simulink model "Five_level_MCI_PMSM_Control_1_fault_tolerant"  (R2025a)
settings: Solver=VariableStepAuto  StartTime=0.0  StopTime=13  RelTol=1e-3
undefined symbols (not defined in the file or in its folder): Ion, Lithium
libraries: spsIGBTDiodeLib x24, spsCurrentMeasurementLib x12, spsVoltageMeasurementLib x6, spsBatteryLib x6, spsRMSLib x6, spsBreakerLib x4, slpidlib x1, spsGroundLib x1, spsPermanentMagnetSynchronousMachineLib x1, simulink x1, spsThreePhaseVIMeasurementLib x1, sps_lib x1
settings Model: Creator=mugun  LastModifiedBy=mugun

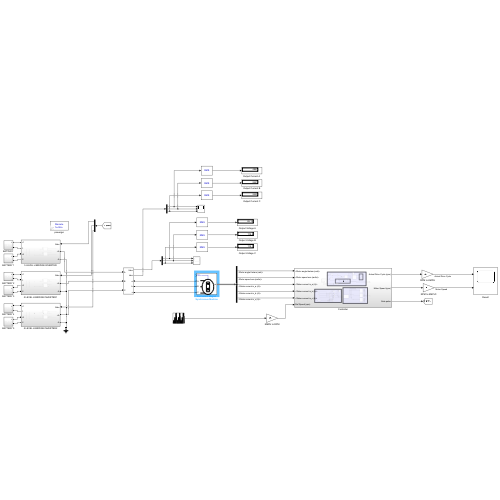
[thumbnail: Simulink's stored preview of the top-level diagram]
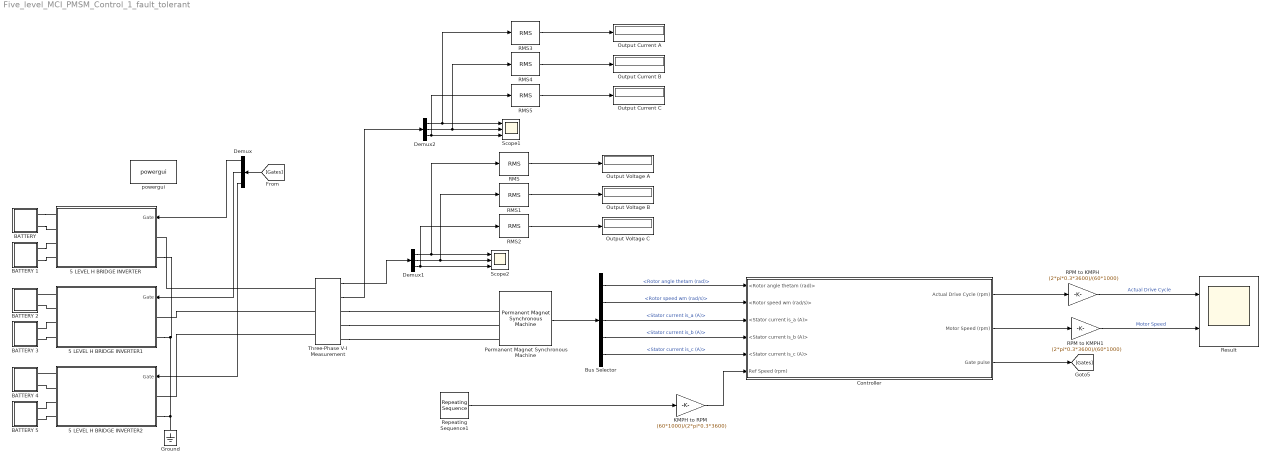
== system Five_level_MCI_PMSM_Control_1_fault_tolerant ==
  5 LEVEL H BRIDGE INVERTER : Subsystem
      settings: PortSchema="{\"entries\":[{\"content\":{\"sides\":[{\"content\":{\"connectorIds\":[\"LConn1\",\"LConn2\",\"LConn3\",\"LConn4\"]},\"type\":\"ConnectorPlacement.EquallySpacedRectSide\",\"uuid\":\"a99ba5a4-868b-4ca9-ae89-158e30df76de\"},{\"content\":{\"connectorIds\":[\"In1\",\"RConn1\",\"RConn2\"],\"side\":\"RIGHT\"},\"type\":\"ConnectorPlacement.EquallySpacedRectSide\",\"uuid\":\"907b6b32-6b28-4f9b-aa63-058c17a50e82\"},{\"content\":{\"side\":\"TOP\"},\"type\":\"ConnectorPlacement.EquallySpacedRectSide\",\"uuid\":\"64bd340d-5502-4b77-92cb-0ed146f38aa8\"}]},\"type\":\"ConnectorPlacement.EquallySpacedConnector\",\"uuid\":\"1fa2cca1-805b-4996-9e9c-123ddddb2b33\"}],\"packageUris\":[\"http://schema.mathworks.com/mf0/Connector/R2020b\"],\"version\":\"1.0\"}"
  5 LEVEL H BRIDGE INVERTER1 : Subsystem
      settings: PortSchema="{\"entries\":[{\"content\":{\"sides\":[{\"content\":{\"connectorIds\":[\"LConn1\",\"LConn2\",\"LConn3\",\"LConn4\"]},\"type\":\"ConnectorPlacement.EquallySpacedRectSide\",\"uuid\":\"a99ba5a4-868b-4ca9-ae89-158e30df76de\"},{\"content\":{\"connectorIds\":[\"In1\",\"RConn1\",\"RConn2\"],\"side\":\"RIGHT\"},\"type\":\"ConnectorPlacement.EquallySpacedRectSide\",\"uuid\":\"907b6b32-6b28-4f9b-aa63-058c17a50e82\"},{\"content\":{\"side\":\"TOP\"},\"type\":\"ConnectorPlacement.EquallySpacedRectSide\",\"uuid\":\"64bd340d-5502-4b77-92cb-0ed146f38aa8\"}]},\"type\":\"ConnectorPlacement.EquallySpacedConnector\",\"uuid\":\"1fa2cca1-805b-4996-9e9c-123ddddb2b33\"}],\"packageUris\":[\"http://schema.mathworks.com/mf0/Connector/R2020b\"],\"version\":\"1.0\"}"
  5 LEVEL H BRIDGE INVERTER2 : Subsystem
      settings: PortSchema="{\"entries\":[{\"content\":{\"sides\":[{\"content\":{\"connectorIds\":[\"LConn1\",\"LConn2\",\"LConn3\",\"LConn4\"]},\"type\":\"ConnectorPlacement.EquallySpacedRectSide\",\"uuid\":\"a99ba5a4-868b-4ca9-ae89-158e30df76de\"},{\"content\":{\"connectorIds\":[\"In1\",\"RConn1\",\"RConn2\"],\"side\":\"RIGHT\"},\"type\":\"ConnectorPlacement.EquallySpacedRectSide\",\"uuid\":\"907b6b32-6b28-4f9b-aa63-058c17a50e82\"},{\"content\":{\"side\":\"TOP\"},\"type\":\"ConnectorPlacement.EquallySpacedRectSide\",\"uuid\":\"64bd340d-5502-4b77-92cb-0ed146f38aa8\"}]},\"type\":\"ConnectorPlacement.EquallySpacedConnector\",\"uuid\":\"1fa2cca1-805b-4996-9e9c-123ddddb2b33\"}],\"packageUris\":[\"http://schema.mathworks.com/mf0/Connector/R2020b\"],\"version\":\"1.0\"}"
  "BATTERY " : Subsystem
  BATTERY 1 : Subsystem
  BATTERY 2 : Subsystem
  BATTERY 3 : Subsystem
  BATTERY 4 : Subsystem
  BATTERY 5 : Subsystem
  Bus Selector : BusSelector  OutputSignals=Rotor angle thetam (rad),Rotor speed wm (rad/s),Stator current is_a (A),Stator current is_b (A),Stator current is_c (A)
  Controller : Subsystem
  Demux : Demux  Outputs=3
  Demux1 : Demux  Outputs=3
  Demux2 : Demux  Outputs=3
  Ground : spsGroundLib/Ground  LConnTagsString=a
  KMPH to RPM : Gain  Gain=(60*1000)/(2*pi*0.3*3600)
  "Output Current A " : Display
  Output Current B : Display
  Output Current C : Display
  Output Voltage A : Display
  Output Voltage B : Display
  Output Voltage C : Display
  Permanent Magnet Synchronous Machine : spsPermanentMagnetSynchronousMachineLib/Permanent Magnet Synchronous Machine  NbPhases=3  FluxDistribution=Sinusoidal  RotorType=Round  MechanicalLoad=Torque Tm  PresetModel=No  ShowDetailedParameters=on  MeasurementBus=off  Resistance=0.02  Inductance=8.5e-3  dqInductances=[8.5e-3,8.5e-3]  La=0.00025  MachineConstant=Flux linkage established by magnets (V.s)  Flux=0.133833  VoltageCst=97.0985  TorqueCst=0.803  Flat=120  Mechanical=[0.008 0.003 4]  PolePairs=4  InitialConditions=[0,0, 0,0]  InitialConditions5ph=[0 0 0 0 0 0]  RefAngle=90 degrees behind phase A axis (modified Park)  IterativeDiscreteModel=Trapezoidal non iterative  TsBlock=-1  TsPowergui=0
  RMS{,1..5} (6 alike) : spsRMSLib/RMS  TrueRMS=on  Freq=60  RMSInit=120  Ts=0
  RPM to KMPH : Gain  Gain=(2*pi*0.3*3600)/(60*1000)
  RPM to KMPH1 : Gain  Gain=(2*pi*0.3*3600)/(60*1000)
  Repeating Sequence1 : simulink/Sources/Repeating Sequence  rep_seq_t=[0 1 2 3 4 5 6 7 8 9 10 11 11.0001 12 13]  rep_seq_y=[0 0 10 10 0 0 20 20 0 0 35 35 25 25 0]
  Result : Scope  NumInputPorts=2
      settings: ActiveDisplayYMinimum=-1  ActiveDisplayYMaximum=1  DataLoggingVariableName=ScopeData8
  Scope1 : Scope  NumInputPorts=3
      settings: ActiveDisplayYMinimum=-1.0013001136517929  ActiveDisplayYMaximum=1.1229859234420478
  Scope2 : Scope  NumInputPorts=3
      settings: ActiveDisplayYMinimum=-132.61800974908385  ActiveDisplayYMaximum=132.61868398150364  DataLoggingVariableName=ScopeData9
  Three-Phase V-I Measurement : spsThreePhaseVIMeasurementLib/Three-Phase V-I Measurement  VoltageMeasurement=phase-to-ground  SetLabelV=off  LabelV=Vabc  Vpu=off  VpuLL=off  CurrentMeasurement=yes  SetLabelI=off  LabelI=Iabc  Ipu=off  Pbase=100e6  Vbase=500e3  OutputType=Complex  PhasorSimulation=off  PSBequivalent=0
  powergui : sps_lib/powergui  Priority=1  SimulationMode=Discrete  SampleTime=1e-6  frequency=60  Iterations=50  frequencyindice=0  Pbase=100e6  ErrMax=1e-4  UnitsV=kV  UnitsW=MW  buscounter=0  FunctionMessages=off  echomessages=off  EnableUseOfTLC=off  CurrentSourceSwitches=off  DisableSnubberDevices=off  DisableRonSwitches=off  DisableVfSwitches=off  DisplayEquations=off  AutomaticDiscreteSolvers=off  SolverType=Tustin/Backward Euler (TBE)  Interpol=off  ExternalGateDelay=off  methode=off  Ts=100  x0status=blocks  SPID=on  SwTol=0  HookPort=off  NonlinearTolerance=1e-4  nMaxIteration=100  ContinueOnMaxIteration=off  RestoreLinks=warning  ResistiveCurrentMeasurement=off  Frange=[0:2:500]  Ylog=off  Xlog=on  ShowGrid=off  save=off  variable=ZData  structure=0  ZoomFFT=off  StartTime=0.0  cycles=1  DisplayStyle=1  fundamental=60  FreqAxis=off  MaxFrequency=1000  frequencyindicesteady=1  RmsSteady=1  display=off
  wires:
  RMS2/1 -> Output Voltage C/1
  KMPH to RPM/1 -> Controller/6(Ref Speed (rpm))
  Bus Selector/3 -> Controller/3(<Stator current is_a (A)>)  "<Stator current is_a (A)>"
  Demux1/1 -> RMS/1, Scope2/1
  Three-Phase V-I Measurement/1 -> Demux1/1
  Demux1/2 -> RMS1/1, Scope2/2
  Demux1/3 -> RMS2/1, Scope2/3
  RMS/1 -> Output Voltage A/1
  Permanent Magnet Synchronous Machine/1 -> Bus Selector/1
  Bus Selector/2 -> Controller/2(<Rotor speed wm (rad/s)>)  "<Rotor speed wm (rad/s)>"
  Bus Selector/4 -> Controller/4(<Stator current is_b (A)>)  "<Stator current is_b (A)>"
  RMS1/1 -> Output Voltage B/1
  Controller/3(Gate pulse) -> [Gates]
  Controller/2(Motor Speed (rpm)) -> RPM to KMPH1/1
  Controller/1(Actual Drive Cycle (rpm)) -> RPM to KMPH/1
  Bus Selector/1 -> Controller/1(<Rotor angle thetam (rad)>)  "<Rotor angle thetam (rad)>"
  Bus Selector/5 -> Controller/5(<Stator current is_c (A)>)  "<Stator current is_c (A)>"
  Demux/1 -> 5 LEVEL H BRIDGE INVERTER/1(Gate)
  Demux/2 -> 5 LEVEL H BRIDGE INVERTER1/1(Gate)
  Demux/3 -> 5 LEVEL H BRIDGE INVERTER2/1(Gate)
  [Gates] -> Demux/1
  RPM to KMPH/1 -> Result/1  "Actual Drive Cycle"
  RPM to KMPH1/1 -> Result/2  "Motor Speed"
  Repeating Sequence1/1 -> KMPH to RPM/1
  RMS3/1 -> "Output Current A "/1
  RMS4/1 -> Output Current B/1
  Demux2/2 -> RMS4/1, Scope1/2
  Demux2/1 -> RMS3/1, Scope1/1
  Demux2/3 -> RMS5/1, Scope1/3
  Three-Phase V-I Measurement/2 -> Demux2/1
  RMS5/1 -> Output Current C/1
  connections:
  Three-Phase V-I Measurement/RConn2 -- Permanent Magnet Synchronous Machine/LConn2
  Three-Phase V-I Measurement/RConn1 -- Permanent Magnet Synchronous Machine/LConn1
  Three-Phase V-I Measurement/RConn3 -- Permanent Magnet Synchronous Machine/LConn3
  Ground/LConn1 -- 5 LEVEL H BRIDGE INVERTER/RConn2 -- 5 LEVEL H BRIDGE INVERTER1/RConn2 -- 5 LEVEL H BRIDGE INVERTER2/RConn2
  5 LEVEL H BRIDGE INVERTER2/LConn4 -- BATTERY 5/LConn2
  5 LEVEL H BRIDGE INVERTER1/LConn1 -- BATTERY 2/LConn1
  5 LEVEL H BRIDGE INVERTER2/LConn1 -- BATTERY 4/LConn1
  BATTERY 1/LConn2 -- 5 LEVEL H BRIDGE INVERTER/LConn4
  5 LEVEL H BRIDGE INVERTER2/LConn3 -- BATTERY 5/LConn1
  5 LEVEL H BRIDGE INVERTER1/LConn3 -- BATTERY 3/LConn1
  5 LEVEL H BRIDGE INVERTER2/LConn2 -- BATTERY 4/LConn2
  Three-Phase V-I Measurement/LConn2 -- 5 LEVEL H BRIDGE INVERTER1/RConn1
  Three-Phase V-I Measurement/LConn3 -- 5 LEVEL H BRIDGE INVERTER2/RConn1
  5 LEVEL H BRIDGE INVERTER1/LConn4 -- BATTERY 3/LConn2
  Three-Phase V-I Measurement/LConn1 -- 5 LEVEL H BRIDGE INVERTER/RConn1
  "BATTERY "/LConn1 -- 5 LEVEL H BRIDGE INVERTER/LConn1
  5 LEVEL H BRIDGE INVERTER1/LConn2 -- BATTERY 2/LConn2
  BATTERY 1/LConn1 -- 5 LEVEL H BRIDGE INVERTER/LConn3
  "BATTERY "/LConn2 -- 5 LEVEL H BRIDGE INVERTER/LConn2

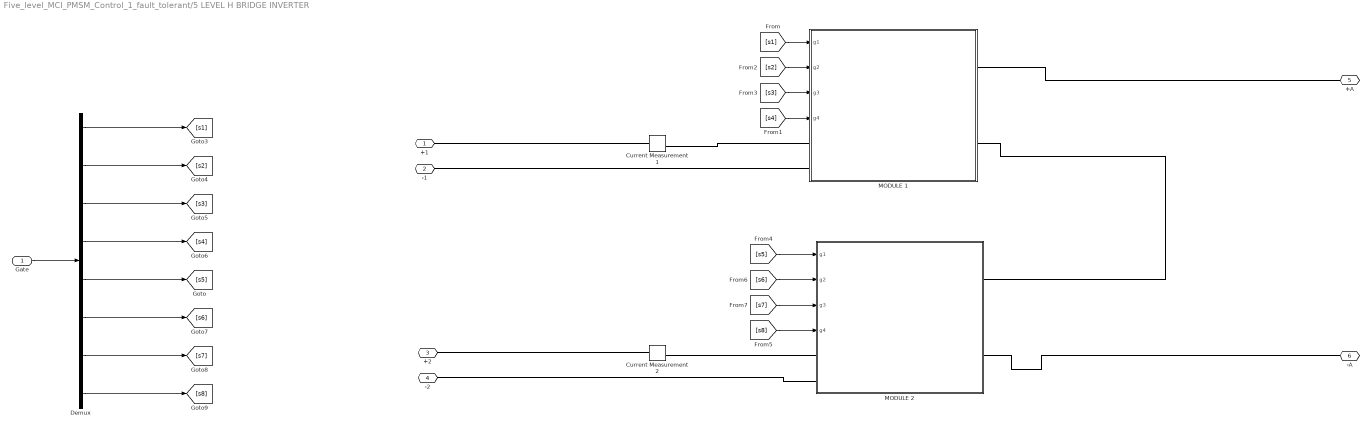
== system Five_level_MCI_PMSM_Control_1_fault_tolerant/5 LEVEL H BRIDGE INVERTER ==
  Gate : Inport
  Current Measurement1 : spsCurrentMeasurementLib/Current Measurement  PhasorSimulation=off  OutputType=Complex  PSBequivalent=0
  Current Measurement2 : spsCurrentMeasurementLib/Current Measurement  PhasorSimulation=off  OutputType=Complex  PSBequivalent=0
  Demux : Demux  Outputs=8
  MODULE 1 : Subsystem
  MODULE 2 : Subsystem
  +1 : PMIOPort  Side=Left
  -1 : PMIOPort  Port=2  Side=Left
  +2 : PMIOPort  Port=3  Side=Left
  -2 : PMIOPort  Port=4  Side=Left
  +A : PMIOPort  Port=5  Side=Right
  -A : PMIOPort  Port=6  Side=Right
  wires:
  Demux/1 -> [s1]
  Demux/2 -> [s2]
  Demux/3 -> [s3]
  Demux/4 -> [s4]
  Demux/5 -> [s5]
  Demux/6 -> [s6]
  Demux/7 -> [s7]
  Demux/8 -> [s8]
  Gate/1 -> Demux/1
  [s3] -> MODULE 1/3(g3)
  [s1] -> MODULE 1/1(g1)
  [s4] -> MODULE 1/4(g4)
  [s2] -> MODULE 1/2(g2)
  [s6] -> MODULE 2/2(g2)
  [s8] -> MODULE 2/4(g4)
  [s5] -> MODULE 2/1(g1)
  [s7] -> MODULE 2/3(g3)
  connections:
  +1/RConn1 -- Current Measurement1/LConn1
  Current Measurement1/RConn1 -- MODULE 1/LConn1
  -1/RConn1 -- MODULE 1/LConn2
  Current Measurement2/RConn1 -- MODULE 2/LConn1
  -2/RConn1 -- MODULE 2/LConn2
  +2/RConn1 -- Current Measurement2/LConn1
  MODULE 1/RConn1 -- +A/RConn1
  MODULE 1/RConn2 -- MODULE 2/RConn1
  MODULE 2/RConn2 -- -A/RConn1

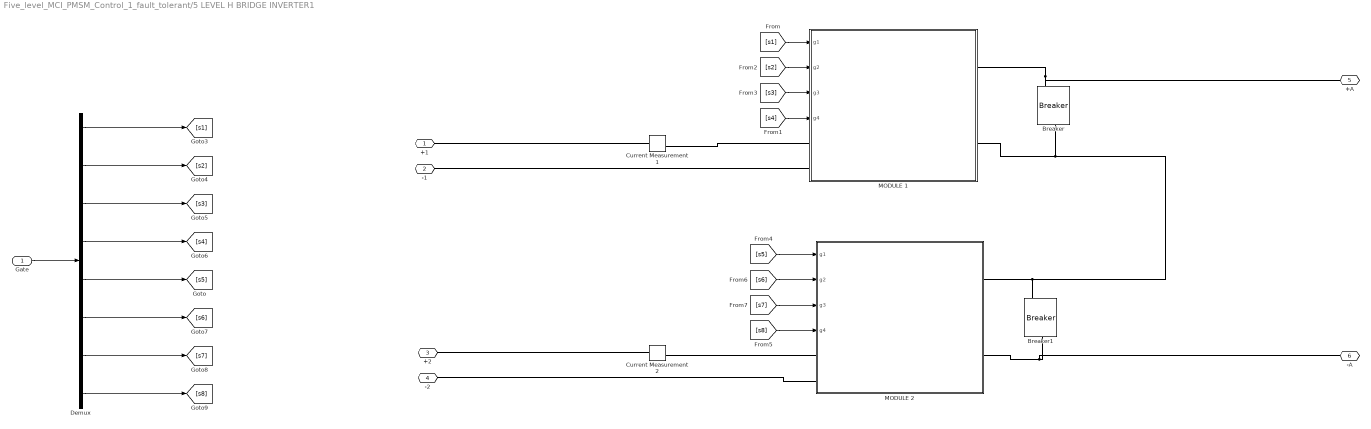
== system Five_level_MCI_PMSM_Control_1_fault_tolerant/5 LEVEL H BRIDGE INVERTER1 ==
  Gate : Inport
  Breaker : spsBreakerLib/Breaker  InitialState=0  SwitchingTimes="[1/60  5/60]"  External=on  BreakerResistance=0.01  SnubberResistance=1e10  SnubberCapacitance=inf  Measurements=None  MoreParameters=on  NoBreakLoop=off
  Breaker1 : spsBreakerLib/Breaker  InitialState=0  SwitchingTimes="[1/60  5/60]"  External=on  BreakerResistance=0.01  SnubberResistance=1e10  SnubberCapacitance=inf  Measurements=None  MoreParameters=on  NoBreakLoop=off
  Current Measurement1 : spsCurrentMeasurementLib/Current Measurement  PhasorSimulation=off  OutputType=Complex  PSBequivalent=0
  Current Measurement2 : spsCurrentMeasurementLib/Current Measurement  PhasorSimulation=off  OutputType=Complex  PSBequivalent=0
  Demux : Demux  Outputs=8
  MODULE 1 : Subsystem
  MODULE 2 : Subsystem
  +1 : PMIOPort  Side=Left
  -1 : PMIOPort  Port=2  Side=Left
  +2 : PMIOPort  Port=3  Side=Left
  -2 : PMIOPort  Port=4  Side=Left
  +A : PMIOPort  Port=5  Side=Right
  -A : PMIOPort  Port=6  Side=Right
  wires:
  Demux/1 -> [s1]
  Demux/2 -> [s2]
  Demux/3 -> [s3]
  Demux/4 -> [s4]
  Demux/5 -> [s5]
  Demux/6 -> [s6]
  Demux/7 -> [s7]
  Demux/8 -> [s8]
  Gate/1 -> Demux/1
  [s3] -> MODULE 1/3(g3)
  [s1] -> MODULE 1/1(g1)
  [s4] -> MODULE 1/4(g4)
  [s2] -> MODULE 1/2(g2)
  [s6] -> MODULE 2/2(g2)
  [s8] -> MODULE 2/4(g4)
  [s5] -> MODULE 2/1(g1)
  [s7] -> MODULE 2/3(g3)
  connections:
  +1/RConn1 -- Current Measurement1/LConn1
  Current Measurement1/RConn1 -- MODULE 1/LConn1
  -1/RConn1 -- MODULE 1/LConn2
  Current Measurement2/RConn1 -- MODULE 2/LConn1
  -2/RConn1 -- MODULE 2/LConn2
  +2/RConn1 -- Current Measurement2/LConn1
  Breaker/RConn1 -- MODULE 1/RConn2 -- MODULE 2/RConn1 -- Breaker1/LConn1
  Breaker1/RConn1 -- -A/RConn1 -- MODULE 2/RConn2
  MODULE 1/RConn1 -- Breaker/LConn1 -- +A/RConn1

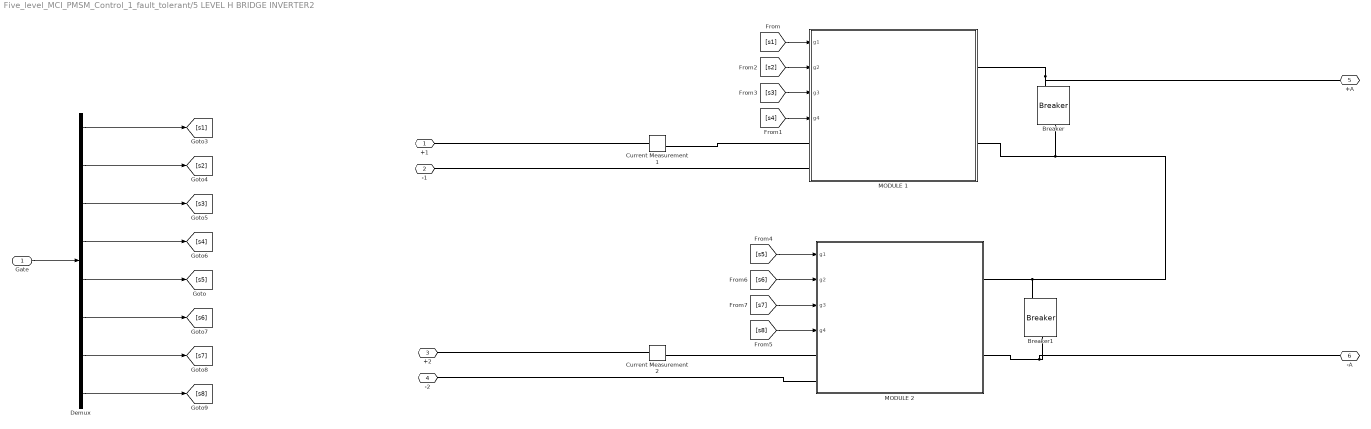
== system Five_level_MCI_PMSM_Control_1_fault_tolerant/5 LEVEL H BRIDGE INVERTER2 ==
  Gate : Inport
  Breaker : spsBreakerLib/Breaker  InitialState=0  SwitchingTimes="[1/60  5/60]"  External=on  BreakerResistance=0.01  SnubberResistance=1e10  SnubberCapacitance=inf  Measurements=None  MoreParameters=on  NoBreakLoop=off
  Breaker1 : spsBreakerLib/Breaker  InitialState=0  SwitchingTimes="[1/60  5/60]"  External=on  BreakerResistance=0.01  SnubberResistance=1e10  SnubberCapacitance=inf  Measurements=None  MoreParameters=on  NoBreakLoop=off
  Current Measurement1 : spsCurrentMeasurementLib/Current Measurement  PhasorSimulation=off  OutputType=Complex  PSBequivalent=0
  Current Measurement2 : spsCurrentMeasurementLib/Current Measurement  PhasorSimulation=off  OutputType=Complex  PSBequivalent=0
  Demux : Demux  Outputs=8
  MODULE 1 : Subsystem
  MODULE 2 : Subsystem
  +1 : PMIOPort  Side=Left
  -1 : PMIOPort  Port=2  Side=Left
  +2 : PMIOPort  Port=3  Side=Left
  -2 : PMIOPort  Port=4  Side=Left
  +A : PMIOPort  Port=5  Side=Right
  -A : PMIOPort  Port=6  Side=Right
  wires:
  Demux/1 -> [s1]
  Demux/2 -> [s2]
  Demux/3 -> [s3]
  Demux/4 -> [s4]
  Demux/5 -> [s5]
  Demux/6 -> [s6]
  Demux/7 -> [s7]
  Demux/8 -> [s8]
  Gate/1 -> Demux/1
  [s3] -> MODULE 1/3(g3)
  [s1] -> MODULE 1/1(g1)
  [s4] -> MODULE 1/4(g4)
  [s2] -> MODULE 1/2(g2)
  [s6] -> MODULE 2/2(g2)
  [s8] -> MODULE 2/4(g4)
  [s5] -> MODULE 2/1(g1)
  [s7] -> MODULE 2/3(g3)
  connections:
  +1/RConn1 -- Current Measurement1/LConn1
  Current Measurement1/RConn1 -- MODULE 1/LConn1
  -1/RConn1 -- MODULE 1/LConn2
  Current Measurement2/RConn1 -- MODULE 2/LConn1
  -2/RConn1 -- MODULE 2/LConn2
  +2/RConn1 -- Current Measurement2/LConn1
  Breaker/RConn1 -- MODULE 1/RConn2 -- MODULE 2/RConn1 -- Breaker1/LConn1
  Breaker1/RConn1 -- -A/RConn1 -- MODULE 2/RConn2
  MODULE 1/RConn1 -- Breaker/LConn1 -- +A/RConn1

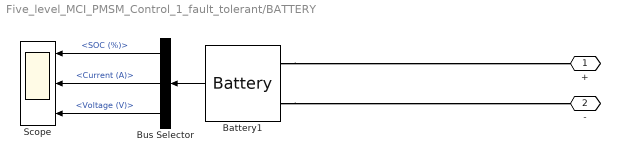
== system Five_level_MCI_PMSM_Control_1_fault_tolerant/BATTERY  ==
  Battery1 : spsBatteryLib/Battery  BatType=Lithium-Ion  NomV=98  NomQ=110  SOC=80  Batt_Tr=0.1  PresetModel=on  MaxQ=110  MinV=73.5  FullV=114.0707  Dis_rate=47.8261  R=0.0089091  Normal_OP=99.4783  expZone="[105.8778      5.404348]"
  Bus Selector : BusSelector  OutputSignals=SOC (%),Current (A),Voltage (V)
  Scope : Scope  NumInputPorts=3
      settings: ActiveDisplayYMinimum=80.6576402320921  ActiveDisplayYMaximum=80.657640232110069
  + : PMIOPort  Side=Left
  - : PMIOPort  Port=2  Side=Left
  wires:
  Bus Selector/3 -> Scope/3  "<Voltage (V)>"
  Battery1/1 -> Bus Selector/1
  Bus Selector/2 -> Scope/2  "<Current (A)>"
  Bus Selector/1 -> Scope/1  "<SOC (%)>"
  connections:
  Battery1/LConn2 -- -/RConn1
  Battery1/LConn1 -- +/RConn1

== system Five_level_MCI_PMSM_Control_1_fault_tolerant/BATTERY 1 ==
  Battery1 : spsBatteryLib/Battery  BatType=Lithium-Ion  NomV=98  NomQ=110  SOC=80  Batt_Tr=0.1  PresetModel=on  MaxQ=110  MinV=73.5  FullV=114.0707  Dis_rate=47.8261  R=0.0089091  Normal_OP=99.4783  expZone="[105.8778      5.404348]"
  Bus Selector : BusSelector  OutputSignals=SOC (%),Current (A),Voltage (V)
  Scope : Scope  NumInputPorts=3
      settings: ActiveDisplayYMinimum=80.6576402320921  ActiveDisplayYMaximum=80.657640232110069
  + : PMIOPort  Side=Left
  - : PMIOPort  Port=2  Side=Left
  wires:
  Bus Selector/3 -> Scope/3  "<Voltage (V)>"
  Battery1/1 -> Bus Selector/1
  Bus Selector/2 -> Scope/2  "<Current (A)>"
  Bus Selector/1 -> Scope/1  "<SOC (%)>"
  connections:
  Battery1/LConn2 -- -/RConn1
  Battery1/LConn1 -- +/RConn1

== system Five_level_MCI_PMSM_Control_1_fault_tolerant/BATTERY 2 ==
  Battery1 : spsBatteryLib/Battery  BatType=Lithium-Ion  NomV=98  NomQ=110  SOC=80  Batt_Tr=0.1  PresetModel=on  MaxQ=110  MinV=73.5  FullV=114.0707  Dis_rate=47.8261  R=0.0089091  Normal_OP=99.4783  expZone="[105.8778      5.404348]"
  Bus Selector : BusSelector  OutputSignals=SOC (%),Current (A),Voltage (V)
  Scope : Scope  NumInputPorts=3
      settings: ActiveDisplayYMinimum=80.6576402320921  ActiveDisplayYMaximum=80.657640232110069
  + : PMIOPort  Side=Left
  - : PMIOPort  Port=2  Side=Left
  wires:
  Bus Selector/3 -> Scope/3  "<Voltage (V)>"
  Battery1/1 -> Bus Selector/1
  Bus Selector/2 -> Scope/2  "<Current (A)>"
  Bus Selector/1 -> Scope/1  "<SOC (%)>"
  connections:
  Battery1/LConn2 -- -/RConn1
  Battery1/LConn1 -- +/RConn1

== system Five_level_MCI_PMSM_Control_1_fault_tolerant/BATTERY 3 ==
  Battery1 : spsBatteryLib/Battery  BatType=Lithium-Ion  NomV=98  NomQ=110  SOC=80  Batt_Tr=0.1  PresetModel=on  MaxQ=110  MinV=73.5  FullV=114.0707  Dis_rate=47.8261  R=0.0089091  Normal_OP=99.4783  expZone="[105.8778      5.404348]"
  Bus Selector : BusSelector  OutputSignals=SOC (%),Current (A),Voltage (V)
  Scope : Scope  NumInputPorts=3
      settings: ActiveDisplayYMinimum=80.6576402320921  ActiveDisplayYMaximum=80.657640232110069
  + : PMIOPort  Side=Left
  - : PMIOPort  Port=2  Side=Left
  wires:
  Bus Selector/3 -> Scope/3  "<Voltage (V)>"
  Battery1/1 -> Bus Selector/1
  Bus Selector/2 -> Scope/2  "<Current (A)>"
  Bus Selector/1 -> Scope/1  "<SOC (%)>"
  connections:
  Battery1/LConn2 -- -/RConn1
  Battery1/LConn1 -- +/RConn1

== system Five_level_MCI_PMSM_Control_1_fault_tolerant/BATTERY 4 ==
  Battery1 : spsBatteryLib/Battery  BatType=Lithium-Ion  NomV=98  NomQ=110  SOC=80  Batt_Tr=0.1  PresetModel=on  MaxQ=110  MinV=73.5  FullV=114.0707  Dis_rate=47.8261  R=0.0089091  Normal_OP=99.4783  expZone="[105.8778      5.404348]"
  Bus Selector : BusSelector  OutputSignals=SOC (%),Current (A),Voltage (V)
  Scope : Scope  NumInputPorts=3
      settings: ActiveDisplayYMinimum=80.6576402320921  ActiveDisplayYMaximum=80.657640232110069
  + : PMIOPort  Side=Left
  - : PMIOPort  Port=2  Side=Left
  wires:
  Bus Selector/3 -> Scope/3  "<Voltage (V)>"
  Battery1/1 -> Bus Selector/1
  Bus Selector/2 -> Scope/2  "<Current (A)>"
  Bus Selector/1 -> Scope/1  "<SOC (%)>"
  connections:
  Battery1/LConn2 -- -/RConn1
  Battery1/LConn1 -- +/RConn1

== system Five_level_MCI_PMSM_Control_1_fault_tolerant/BATTERY 5 ==
  Battery1 : spsBatteryLib/Battery  BatType=Lithium-Ion  NomV=98  NomQ=110  SOC=80  Batt_Tr=0.1  PresetModel=on  MaxQ=110  MinV=73.5  FullV=114.0707  Dis_rate=47.8261  R=0.0089091  Normal_OP=99.4783  expZone="[105.8778      5.404348]"
  Bus Selector : BusSelector  OutputSignals=SOC (%),Current (A),Voltage (V)
  Scope : Scope  NumInputPorts=3
      settings: ActiveDisplayYMinimum=80.6576402320921  ActiveDisplayYMaximum=80.657640232110069
  + : PMIOPort  Side=Left
  - : PMIOPort  Port=2  Side=Left
  wires:
  Bus Selector/3 -> Scope/3  "<Voltage (V)>"
  Battery1/1 -> Bus Selector/1
  Bus Selector/2 -> Scope/2  "<Current (A)>"
  Bus Selector/1 -> Scope/1  "<SOC (%)>"
  connections:
  Battery1/LConn2 -- -/RConn1
  Battery1/LConn1 -- +/RConn1

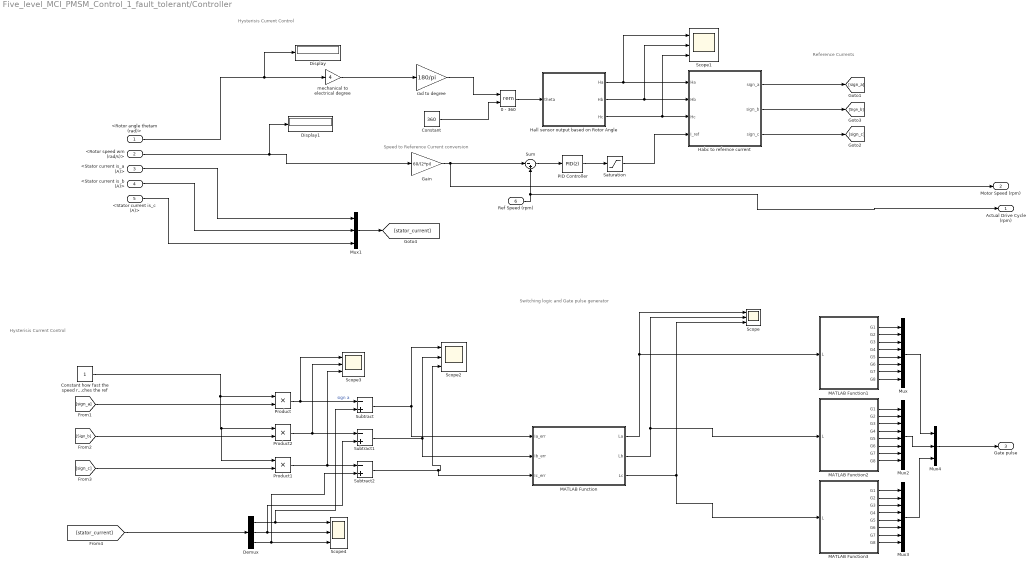
== system Five_level_MCI_PMSM_Control_1_fault_tolerant/Controller ==
  note: Switching logic and Gate pulse generator
  note: Hysterisis Current Control
  note: Hysterisis Current Control
  note: Speed to Reference Current conversion
  note: Reference Currents
  <Rotor angle thetam (rad)> : Inport
  <Rotor speed wm (rad/s)> : Inport  Port=2
  <Stator current is_a (A)> : Inport  Port=3
  <Stator current is_b (A)> : Inport  Port=4
  <Stator current is_c (A)> : Inport  Port=5
  Ref Speed (rpm) : Inport  Port=6
  0 - 360 : Math  Operator=rem
  Constant : Constant  Value=360
  Constant how fast the speed reaches the ref : Constant
  Demux : Demux  Outputs=3
  Display : Display
  Display1 : Display
  Gain : Gain  Gain=60/(2*pi)
  Habc to refernce current : MATLAB Function  TreatAsAtomicUnit=on
  Hall sensor output based on Rotor Angle : MATLAB Function  TreatAsAtomicUnit=on
  MATLAB Function : MATLAB Function  TreatAsAtomicUnit=on
  MATLAB Function1 : MATLAB Function  TreatAsAtomicUnit=on
  MATLAB Function2 : MATLAB Function  TreatAsAtomicUnit=on
  MATLAB Function3 : MATLAB Function  TreatAsAtomicUnit=on
  Mux : Mux  Inputs=8
  Mux1 : Mux  Inputs=3
  Mux2 : Mux  Inputs=8
  Mux3 : Mux  Inputs=8
  Mux4 : Mux  Inputs=3
  PID Controller : slpidlib/PID Controller  Controller=PID  Form=Parallel  TimeDomain=Discrete-time  UseExternalTs=off  SampleTime=-1  IntegratorMethod=Forward Euler  FilterMethod=Forward Euler  ControllerParametersSource=internal  P=1  I=1  UseKiTs=off  D=0  UseExternalDerivativeSource=off  N=100  UseFilter=on  TunerSelectOption=Transfer Function Based (PID Tuner App)  InitialConditionSource=internal  InitialConditionForIntegrator=0  InitialConditionForFilter=0  DifferentiatorICPrevScaledInput=0  ExternalReset=none  TrackingMode=off  Kt=1  LimitOutput=on  SatLimitsSource=internal  UpperSaturationLimit=36.38  LowerSaturationLimit=-36.38  LinearizeAsGain=on  AntiWindupMode=none  Kb=1  LimitIntegrator=off  UpperIntegratorSaturationLimit=inf  LowerIntegratorSaturationLimit=-inf  POutMin=[]  POutMax=[]  IOutMin=[]  IOutMax=[]  DOutMin=[]  DOutMax=[]  NOutMin=[]  NOutMax=[]  SumOutMin=[]  SumOutMax=[]  SaturationOutMin=[]  SaturationOutMax=[]  PParamMin=[]  PParamMax=[]  IParamMin=[]  IParamMax=[]  DParamMin=[]  DParamMax=[]  NParamMin=[]  NParamMax=[]  KbParamMin=[]  KbParamMax=[]  KtParamMin=[]  KtParamMax=[]  KbOutMin=[]  KbOutMax=[]  KtOutMin=[]  KtOutMax=[]  IntegratorOutMin=[]  IntegratorOutMax=[]  FilterOutMin=[]  FilterOutMax=[]  SumI1OutMin=[]  SumI1OutMax=[]  SumI2OutMin=[]  SumI2OutMax=[]  SumI3OutMin=[]  SumI3OutMax=[]  SumI4OutMin=[]  SumI4OutMax=[]  SumDOutMin=[]  SumDOutMax=[]  DifferentiatorOutMin=[]  DifferentiatorOutMax=[]  FilterDiffOutCoefMin=[]  FilterDiffOutCoefMax=[]  ReciprocalOutMin=[]  ReciprocalOutMax=[]  SumDenOutMin=[]  SumDenOutMax=[]  SumNumOutMin=[]  SumNumOutMax=[]  DivideOutMin=[]  DivideOutMax=[]  UdiffTsProdOutMin=[]  UdiffTsProdOutMax=[]  NTsProdOutMin=[]  NTsProdOutMax=[]  UintegralTsProdOutMin=[]  UintegralTsProdOutMax=[]  UngainTsProdOutMin=[]  UngainTsProdOutMax=[]  ClampingZeroOutDataTypeStr=Inherit: Inherit via back propagation  ClampingZeroOutMin=[]  ClampingZeroOutMax=[]  FilterDenConstantOutDataTypeStr=Inherit: Inherit via back propagation  FilterDenConstantOutMin=[]  FilterDenConstantOutMax=[]  PCopyOutDataTypeStr=Inherit: Inherit via back propagation  PCopyOutMin=[]  PCopyOutMax=[]  NCopyOutDataTypeStr=Inherit: Inherit via back propagation  NCopyOutMin=[]  NCopyOutMax=[]  IntegratorContinuousStateAttributes=''  IntegratorStateMustResolveToSignalObject=off  IntegratorRTWStateStorageClass=Auto  FilterContinuousStateAttributes=''  FilterStateMustResolveToSignalObject=off  FilterRTWStateStorageClass=Auto  ParallelPVariant=InternalParameters  IdealPVariant=Disabled  IVariant=InternalParameters  DVariant=InternalParameters  IntegratorVariant=Discrete  SatVariant=Enabled  AWVariant=Passthrough  PCopyVariant=Disabled  TRVariant=Disabled  FdbkBlocksVariant=Forward  IdealPFdbkVariant=Disabled  SatFdbkVariant=Disabled  DerivativeFilterVariant=ForwardEulerFilter  NVariant=InternalParameters  NCopyVariant=Disabled  FilterICVariant=InternalICsFilter  IntegratorICVariant=InternalICs  ExternalResetVariant=Disabled  TRSumVariant=Passthrough  SumFdbkVariant=Disabled  SumVariant=Sum_PID  TsampFilterVariant=InternalTs  TsampNgainVariant=Passthrough  TsampIntegralVariant=Disabled_SignalSpec  ExternalSaturationOutDataTypeStr=Inherit: Same as second input  DerivativeSourceVariant=ErrorSignal  PreIntVariant=InternalPreInt
  Product : Product
  Product1 : Product
  Product2 : Product
  Saturation : Saturate  UpperLimit=73.36  LowerLimit=-73.36
  Scope{,1..4} (5 alike) : Scope  NumInputPorts=3
      Scope settings: ActiveDisplayYMinimum=-2.5  ActiveDisplayYMaximum=2.5
      Scope1 settings: ActiveDisplayYMinimum=-0.12499999999999997  ActiveDisplayYMaximum=1.125  DataLoggingVariableName=ScopeData4
      Scope2 settings: ActiveDisplayYMinimum=-1.5537772622772938  ActiveDisplayYMaximum=1.2440514814341237  DataLoggingVariableName=ScopeData6
      Scope3 settings: ActiveDisplayYMinimum=-3.2408539083396524  ActiveDisplayYMaximum=8.44453932314885  DataLoggingVariableName=ScopeData5
      Scope4 settings: ActiveDisplayYMinimum=-1.1823058707589256  ActiveDisplayYMaximum=1.1505926602747607  DataLoggingVariableName=ScopeData7
  Subtract : Sum  Inputs=-+
  Subtract1 : Sum  Inputs=-+
  Subtract2 : Sum  Inputs=-+
  Sum : Sum  Inputs=|-+
  mechanical to electrical degree : Gain  Gain=4
  rad to degree : Gain  Gain=180/pi
  Actual Drive Cycle (rpm) : Outport
  Motor Speed (rpm) : Outport  Port=2
  Gate pulse : Outport  Port=3
  wires:
  Constant/1 -> 0 - 360/2
  Demux/3 -> Scope4/3, Subtract2/2
  Demux/1 -> Scope4/1, Subtract/2
  <Rotor angle thetam (rad)>/1 -> Display/1, mechanical to electrical degree/1
  <Rotor speed wm (rad/s)>/1 -> Display1/1, Gain/1
  Constant how fast the speed reaches the ref/1 -> Product1/1, Product2/1, Product/1
  Habc to refernce current/2(sign_b) -> [Sign_b]
  rad to degree/1 -> 0 - 360/1
  Hall sensor output based on Rotor Angle/3(Hc) -> Scope1/3, Habc to refernce current/3(Hc)
  [sign_c] -> Product1/2
  Product/1 -> Scope3/1, Subtract/1  "sign a"
  [stator_current] -> Demux/1
  Habc to refernce current/3(sign_c) -> [sign_c]
  Gain/1 -> Motor Speed (rpm)/1, Sum/1
  Hall sensor output based on Rotor Angle/2(Hb) -> Scope1/2, Habc to refernce current/2(Hb)
  Sum/1 -> PID Controller/1
  Demux/2 -> Scope4/2, Subtract1/2
  Product1/1 -> Scope3/3, Subtract2/1
  mechanical to electrical degree/1 -> rad to degree/1
  Habc to refernce current/1(sign_a) -> [sign_a]
  0 - 360/1 -> Hall sensor output based on Rotor Angle/1(theta)
  Mux1/1 -> [stator_current]
  [Sign_b] -> Product2/2
  [sign_a] -> Product/2
  Saturation/1 -> Habc to refernce current/4(I_ref)
  Product2/1 -> Scope3/2, Subtract1/1
  <Stator current is_a (A)>/1 -> Mux1/1
  PID Controller/1 -> Saturation/1
  Hall sensor output based on Rotor Angle/1(Ha) -> Scope1/1, Habc to refernce current/1(Ha)
  <Stator current is_c (A)>/1 -> Mux1/3
  Ref Speed (rpm)/1 -> Actual Drive Cycle (rpm)/1, Sum/2
  <Stator current is_b (A)>/1 -> Mux1/2
  Subtract/1 -> Scope2/1, MATLAB Function/1(Ia_err)
  Subtract1/1 -> Scope2/2, MATLAB Function/2(Ib_err)
  Subtract2/1 -> MATLAB Function/3(Ic_err), Scope2/3
  MATLAB Function/1(La) -> Scope/1, MATLAB Function1/1(L)
  Mux4/1 -> Gate pulse/1
  Mux/1 -> Mux4/1
  MATLAB Function1/1(G1) -> Mux/1
  MATLAB Function1/2(G2) -> Mux/2
  MATLAB Function1/3(G3) -> Mux/3
  MATLAB Function1/4(G4) -> Mux/4
  MATLAB Function1/5(G5) -> Mux/5
  MATLAB Function1/6(G6) -> Mux/6
  MATLAB Function1/7(G7) -> Mux/7
  MATLAB Function1/8(G8) -> Mux/8
  MATLAB Function2/7(G7) -> Mux2/7
  MATLAB Function2/4(G4) -> Mux2/4
  MATLAB Function2/6(G6) -> Mux2/6
  MATLAB Function2/8(G8) -> Mux2/8
  MATLAB Function2/2(G2) -> Mux2/2
  MATLAB Function2/1(G1) -> Mux2/1
  MATLAB Function2/3(G3) -> Mux2/3
  MATLAB Function2/5(G5) -> Mux2/5
  MATLAB Function3/7(G7) -> Mux3/7
  MATLAB Function3/4(G4) -> Mux3/4
  MATLAB Function3/6(G6) -> Mux3/6
  MATLAB Function3/8(G8) -> Mux3/8
  MATLAB Function3/2(G2) -> Mux3/2
  MATLAB Function3/1(G1) -> Mux3/1
  MATLAB Function3/3(G3) -> Mux3/3
  MATLAB Function3/5(G5) -> Mux3/5
  Mux2/1 -> Mux4/2
  Mux3/1 -> Mux4/3
  MATLAB Function/2(Lb) -> Scope/2, MATLAB Function2/1(L)
  MATLAB Function/3(Lc) -> Scope/3, MATLAB Function3/1(L)

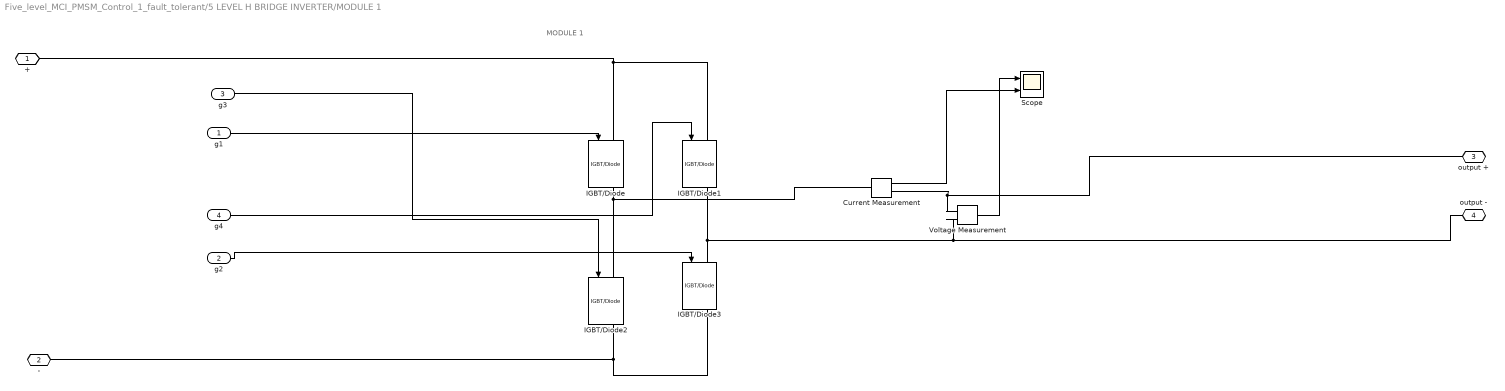
== system Five_level_MCI_PMSM_Control_1_fault_tolerant/5 LEVEL H BRIDGE INVERTER/MODULE 1 ==
  note: MODULE 1
  g1 : Inport
  g2 : Inport  Port=2
  g3 : Inport  Port=3
  g4 : Inport  Port=4
  Current Measurement : spsCurrentMeasurementLib/Current Measurement  PhasorSimulation=off  OutputType=Complex  PSBequivalent=0
  IGBT/Diode{,1..3} (4 alike) : spsIGBTDiodeLib/IGBT//Diode  Ron=1e-3  Rs=1e5  Cs=inf  Measurements=on
  Scope : Scope  NumInputPorts=2
      settings: ActiveDisplayYMinimum=-67.656399857092211  ActiveDisplayYMaximum=67.656345987022974  DataLoggingVariableName=ScopeData2
  Voltage Measurement : spsVoltageMeasurementLib/Voltage Measurement  PhasorSimulation=off  OutputType=Complex  PSBequivalent=0
  + : PMIOPort  Side=Left
  - : PMIOPort  Port=2  Side=Left
  output + : PMIOPort  Port=3  Side=Right
  output - : PMIOPort  Port=4  Side=Right
  wires:
  g1/1 -> IGBT/Diode/1
  Voltage Measurement/1 -> Scope/1
  Current Measurement/1 -> Scope/2
  g2/1 -> IGBT/Diode3/1
  g3/1 -> IGBT/Diode2/1
  g4/1 -> IGBT/Diode1/1
  connections:
  IGBT/Diode/RConn1 -- IGBT/Diode2/LConn1 -- Current Measurement/LConn1
  IGBT/Diode1/RConn1 -- IGBT/Diode3/LConn1 -- Voltage Measurement/LConn2 -- output -/RConn1
  IGBT/Diode3/RConn1 -- -/RConn1 -- IGBT/Diode2/RConn1
  IGBT/Diode/LConn1 -- +/RConn1 -- IGBT/Diode1/LConn1
  Voltage Measurement/LConn1 -- Current Measurement/RConn1 -- output +/RConn1

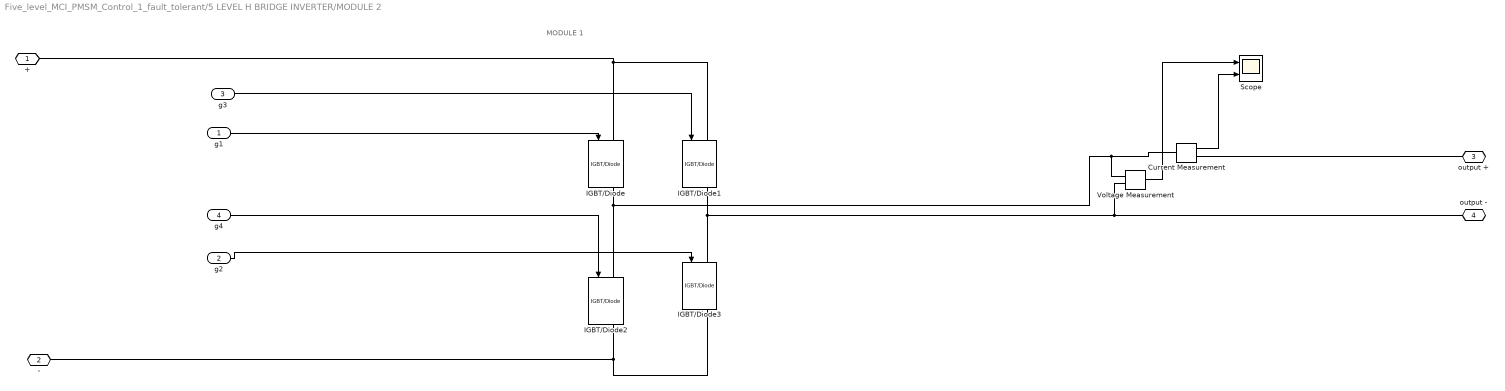
== system Five_level_MCI_PMSM_Control_1_fault_tolerant/5 LEVEL H BRIDGE INVERTER/MODULE 2 ==
  note: MODULE 1
  g1 : Inport
  g2 : Inport  Port=2
  g3 : Inport  Port=3
  g4 : Inport  Port=4
  Current Measurement : spsCurrentMeasurementLib/Current Measurement  PhasorSimulation=off  OutputType=Complex  PSBequivalent=0
  IGBT/Diode{,1..3} (4 alike) : spsIGBTDiodeLib/IGBT//Diode  Ron=1e-3  Rs=1e5  Cs=inf  Measurements=on
  Scope : Scope  NumInputPorts=2
      settings: ActiveDisplayYMinimum=-68.11449112775864  ActiveDisplayYMaximum=67.198291734216028  DataLoggingVariableName=ScopeData3
  Voltage Measurement : spsVoltageMeasurementLib/Voltage Measurement  PhasorSimulation=off  OutputType=Complex  PSBequivalent=0
  + : PMIOPort  Side=Left
  - : PMIOPort  Port=2  Side=Left
  output + : PMIOPort  Port=3  Side=Right
  output - : PMIOPort  Port=4  Side=Right
  wires:
  g1/1 -> IGBT/Diode/1
  Voltage Measurement/1 -> Scope/1
  Current Measurement/1 -> Scope/2
  g2/1 -> IGBT/Diode3/1
  g4/1 -> IGBT/Diode2/1
  g3/1 -> IGBT/Diode1/1
  connections:
  IGBT/Diode/RConn1 -- Voltage Measurement/LConn1 -- Current Measurement/LConn1 -- IGBT/Diode2/LConn1
  IGBT/Diode1/RConn1 -- Voltage Measurement/LConn2 -- output -/RConn1 -- IGBT/Diode3/LConn1
  IGBT/Diode3/RConn1 -- IGBT/Diode2/RConn1 -- -/RConn1
  IGBT/Diode/LConn1 -- IGBT/Diode1/LConn1 -- +/RConn1
  Current Measurement/RConn1 -- output +/RConn1

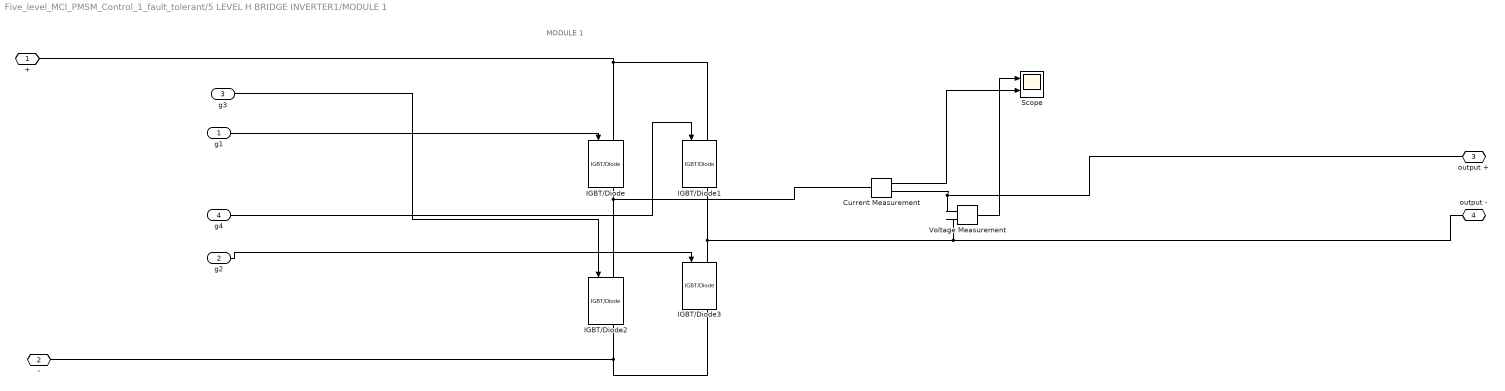
== system Five_level_MCI_PMSM_Control_1_fault_tolerant/5 LEVEL H BRIDGE INVERTER1/MODULE 1 ==
  note: MODULE 1
  g1 : Inport
  g2 : Inport  Port=2
  g3 : Inport  Port=3
  g4 : Inport  Port=4
  Current Measurement : spsCurrentMeasurementLib/Current Measurement  PhasorSimulation=off  OutputType=Complex  PSBequivalent=0
  IGBT/Diode{,1..3} (4 alike) : spsIGBTDiodeLib/IGBT//Diode  Ron=1e-3  Rs=1e5  Cs=inf  Measurements=on
  Scope : Scope  NumInputPorts=2
      settings: ActiveDisplayYMinimum=-67.656399857092211  ActiveDisplayYMaximum=67.656345987022974  DataLoggingVariableName=ScopeData2
  Voltage Measurement : spsVoltageMeasurementLib/Voltage Measurement  PhasorSimulation=off  OutputType=Complex  PSBequivalent=0
  + : PMIOPort  Side=Left
  - : PMIOPort  Port=2  Side=Left
  output + : PMIOPort  Port=3  Side=Right
  output - : PMIOPort  Port=4  Side=Right
  wires:
  g1/1 -> IGBT/Diode/1
  Voltage Measurement/1 -> Scope/1
  Current Measurement/1 -> Scope/2
  g2/1 -> IGBT/Diode3/1
  g3/1 -> IGBT/Diode2/1
  g4/1 -> IGBT/Diode1/1
  connections:
  IGBT/Diode/RConn1 -- IGBT/Diode2/LConn1 -- Current Measurement/LConn1
  IGBT/Diode1/RConn1 -- IGBT/Diode3/LConn1 -- Voltage Measurement/LConn2 -- output -/RConn1
  IGBT/Diode3/RConn1 -- -/RConn1 -- IGBT/Diode2/RConn1
  IGBT/Diode/LConn1 -- +/RConn1 -- IGBT/Diode1/LConn1
  Voltage Measurement/LConn1 -- Current Measurement/RConn1 -- output +/RConn1

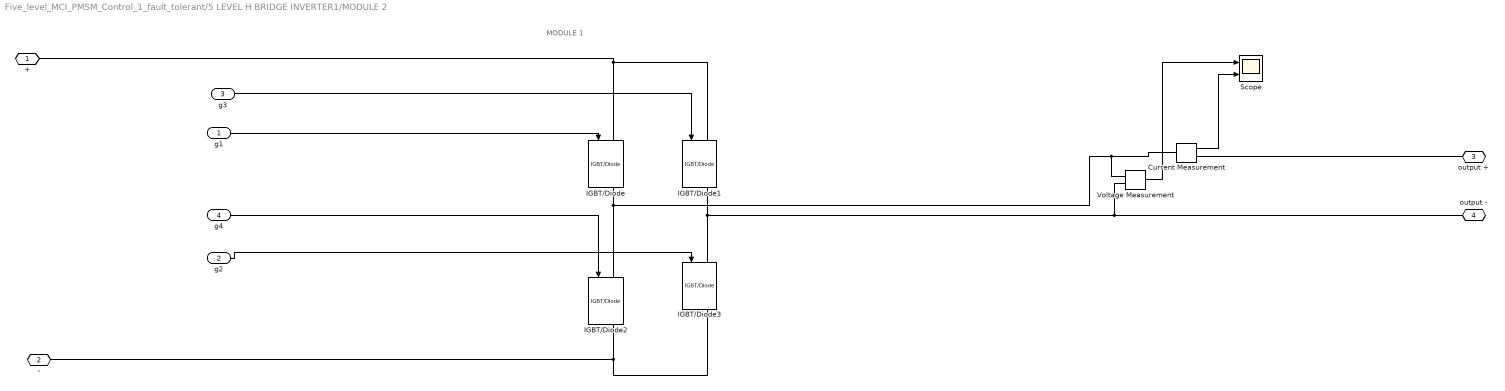
== system Five_level_MCI_PMSM_Control_1_fault_tolerant/5 LEVEL H BRIDGE INVERTER1/MODULE 2 ==
  note: MODULE 1
  g1 : Inport
  g2 : Inport  Port=2
  g3 : Inport  Port=3
  g4 : Inport  Port=4
  Current Measurement : spsCurrentMeasurementLib/Current Measurement  PhasorSimulation=off  OutputType=Complex  PSBequivalent=0
  IGBT/Diode{,1..3} (4 alike) : spsIGBTDiodeLib/IGBT//Diode  Ron=1e-3  Rs=1e5  Cs=inf  Measurements=on
  Scope : Scope  NumInputPorts=2
      settings: ActiveDisplayYMinimum=-68.11449112775864  ActiveDisplayYMaximum=67.198291734216028  DataLoggingVariableName=ScopeData3
  Voltage Measurement : spsVoltageMeasurementLib/Voltage Measurement  PhasorSimulation=off  OutputType=Complex  PSBequivalent=0
  + : PMIOPort  Side=Left
  - : PMIOPort  Port=2  Side=Left
  output + : PMIOPort  Port=3  Side=Right
  output - : PMIOPort  Port=4  Side=Right
  wires:
  g1/1 -> IGBT/Diode/1
  Voltage Measurement/1 -> Scope/1
  Current Measurement/1 -> Scope/2
  g2/1 -> IGBT/Diode3/1
  g4/1 -> IGBT/Diode2/1
  g3/1 -> IGBT/Diode1/1
  connections:
  IGBT/Diode/RConn1 -- Voltage Measurement/LConn1 -- Current Measurement/LConn1 -- IGBT/Diode2/LConn1
  IGBT/Diode1/RConn1 -- Voltage Measurement/LConn2 -- output -/RConn1 -- IGBT/Diode3/LConn1
  IGBT/Diode3/RConn1 -- IGBT/Diode2/RConn1 -- -/RConn1
  IGBT/Diode/LConn1 -- IGBT/Diode1/LConn1 -- +/RConn1
  Current Measurement/RConn1 -- output +/RConn1

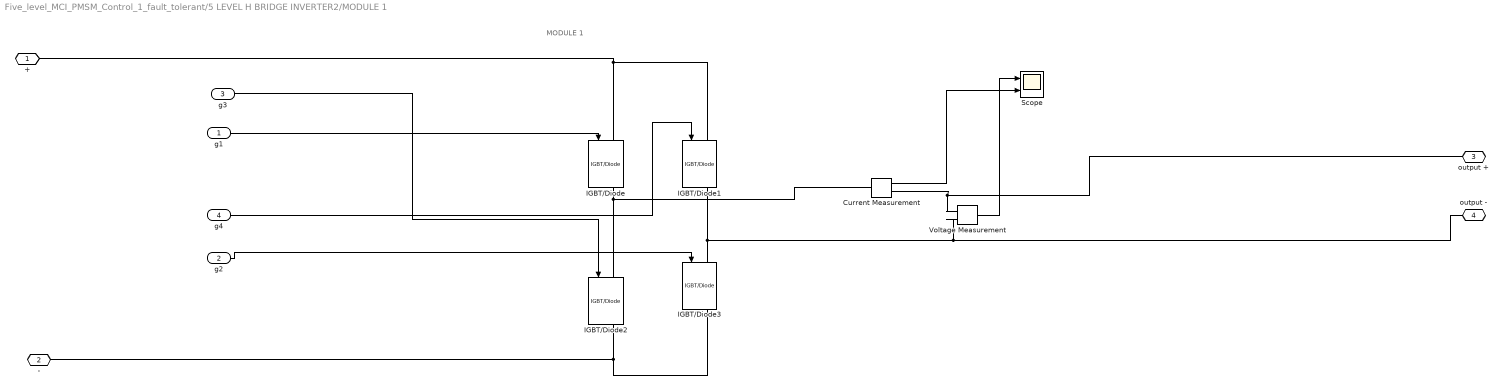
== system Five_level_MCI_PMSM_Control_1_fault_tolerant/5 LEVEL H BRIDGE INVERTER2/MODULE 1 ==
  note: MODULE 1
  g1 : Inport
  g2 : Inport  Port=2
  g3 : Inport  Port=3
  g4 : Inport  Port=4
  Current Measurement : spsCurrentMeasurementLib/Current Measurement  PhasorSimulation=off  OutputType=Complex  PSBequivalent=0
  IGBT/Diode{,1..3} (4 alike) : spsIGBTDiodeLib/IGBT//Diode  Ron=1e-3  Rs=1e5  Cs=inf  Measurements=on
  Scope : Scope  NumInputPorts=2
      settings: ActiveDisplayYMinimum=-67.656399857092211  ActiveDisplayYMaximum=67.656345987022974  DataLoggingVariableName=ScopeData2
  Voltage Measurement : spsVoltageMeasurementLib/Voltage Measurement  PhasorSimulation=off  OutputType=Complex  PSBequivalent=0
  + : PMIOPort  Side=Left
  - : PMIOPort  Port=2  Side=Left
  output + : PMIOPort  Port=3  Side=Right
  output - : PMIOPort  Port=4  Side=Right
  wires:
  g1/1 -> IGBT/Diode/1
  Voltage Measurement/1 -> Scope/1
  Current Measurement/1 -> Scope/2
  g2/1 -> IGBT/Diode3/1
  g3/1 -> IGBT/Diode2/1
  g4/1 -> IGBT/Diode1/1
  connections:
  IGBT/Diode/RConn1 -- IGBT/Diode2/LConn1 -- Current Measurement/LConn1
  IGBT/Diode1/RConn1 -- IGBT/Diode3/LConn1 -- Voltage Measurement/LConn2 -- output -/RConn1
  IGBT/Diode3/RConn1 -- -/RConn1 -- IGBT/Diode2/RConn1
  IGBT/Diode/LConn1 -- +/RConn1 -- IGBT/Diode1/LConn1
  Voltage Measurement/LConn1 -- Current Measurement/RConn1 -- output +/RConn1

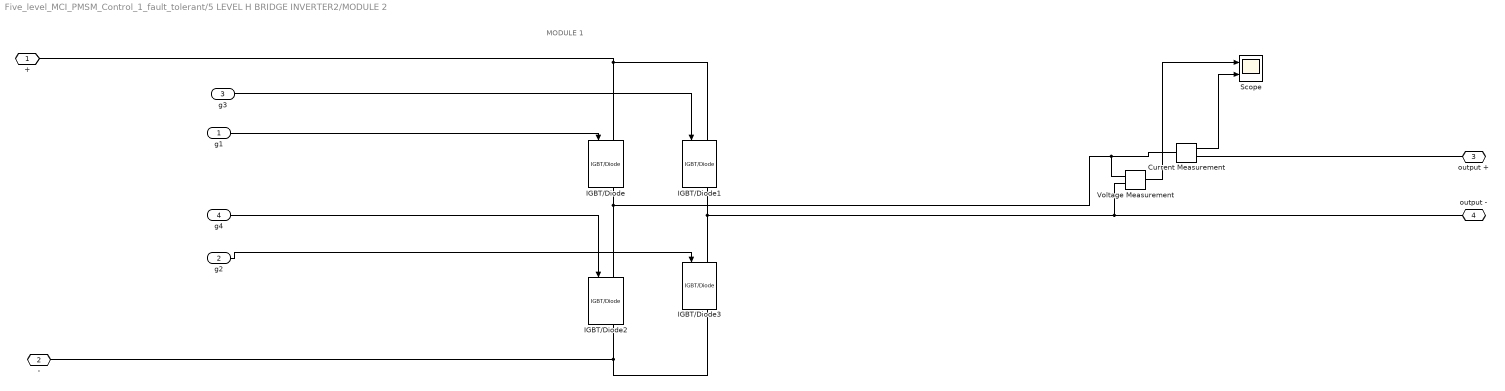
== system Five_level_MCI_PMSM_Control_1_fault_tolerant/5 LEVEL H BRIDGE INVERTER2/MODULE 2 ==
  note: MODULE 1
  g1 : Inport
  g2 : Inport  Port=2
  g3 : Inport  Port=3
  g4 : Inport  Port=4
  Current Measurement : spsCurrentMeasurementLib/Current Measurement  PhasorSimulation=off  OutputType=Complex  PSBequivalent=0
  IGBT/Diode{,1..3} (4 alike) : spsIGBTDiodeLib/IGBT//Diode  Ron=1e-3  Rs=1e5  Cs=inf  Measurements=on
  Scope : Scope  NumInputPorts=2
      settings: ActiveDisplayYMinimum=-68.11449112775864  ActiveDisplayYMaximum=67.198291734216028  DataLoggingVariableName=ScopeData3
  Voltage Measurement : spsVoltageMeasurementLib/Voltage Measurement  PhasorSimulation=off  OutputType=Complex  PSBequivalent=0
  + : PMIOPort  Side=Left
  - : PMIOPort  Port=2  Side=Left
  output + : PMIOPort  Port=3  Side=Right
  output - : PMIOPort  Port=4  Side=Right
  wires:
  g1/1 -> IGBT/Diode/1
  Voltage Measurement/1 -> Scope/1
  Current Measurement/1 -> Scope/2
  g2/1 -> IGBT/Diode3/1
  g4/1 -> IGBT/Diode2/1
  g3/1 -> IGBT/Diode1/1
  connections:
  IGBT/Diode/RConn1 -- Voltage Measurement/LConn1 -- Current Measurement/LConn1 -- IGBT/Diode2/LConn1
  IGBT/Diode1/RConn1 -- Voltage Measurement/LConn2 -- output -/RConn1 -- IGBT/Diode3/LConn1
  IGBT/Diode3/RConn1 -- IGBT/Diode2/RConn1 -- -/RConn1
  IGBT/Diode/LConn1 -- IGBT/Diode1/LConn1 -- +/RConn1
  Current Measurement/RConn1 -- output +/RConn1

== matlab function Five_level_MCI_PMSM_Control_1_fault_tolerant/Controller/Habc to refernce current ==
  data: Ha input; sign_a output; Hb input; Hc input; sign_b output; sign_c output; I_ref input
function [sign_a,sign_b,sign_c] = fcn(Ha,Hb,Hc,I_ref)

if (Ha==1 && Hb==0 && Hc==1)
    sign_a=I_ref;
    sign_b=0;
    sign_c=-I_ref;

elseif (Ha==1 && Hb==0 && Hc==0)
    sign_a=0;
    sign_b=I_ref;
    sign_c=-I_ref;

elseif (Ha==1 && Hb==1 && Hc==0)
    sign_a=-I_ref;
    sign_b=I_ref;
    sign_c=0;

elseif (Ha==0 && Hb==1 && Hc==0)
    sign_a=-I_ref;
    sign_b=0;
    sign_c=I_ref;

elseif (Ha==0 && Hb==1 && Hc==1)
    sign_a=0;
    sign_b=-I_ref;
    sign_c=I_ref;

elseif (Ha==0 && Hb==0 && Hc==1)
    sign_a=I_ref;
    sign_b=-I_ref;
    sign_c=0;

else 
    sign_a=0;
    sign_b=0;
    sign_c=0;

end

== matlab function Five_level_MCI_PMSM_Control_1_fault_tolerant/Controller/MATLAB Function ==
  data: Ia_err input; La output; Lb output; Lc output; Ib_err input; Ic_err input
function [La,Lb,Lc] = MLH7_Controller(Ia_err,Ib_err,Ic_err)
% Multilevel hysteresis controller for 7-level inverter
% Inputs: phase current errors (A)
% Outputs: quantized level commands (-3..+3)
% Author: Rajagopal & ChatGPT (MCI Project)

% --- Tunable hysteresis thresholds (adjust as needed) ---
Delta1 = 1*0.2;   % inner band (A)
Delta2 = 1*0.5;   % mid band (A)


% Compute level for each phase
La = getLevel(Ia_err, Delta1, Delta2);
Lb = getLevel(Ib_err, Delta1, Delta2);
Lc = getLevel(Ic_err, Delta1, Delta2);


end

function L = getLevel(err, D1, D2)
% Converts current error to level command

if err > D2
    L = -2;
elseif err > D1
    L = -1;
elseif err >= -D1 && err <= D1
    L = 0;
elseif err >= -D2
    L = 1;
else
    L = 2;
end

end

== matlab function Five_level_MCI_PMSM_Control_1_fault_tolerant/Controller/Hall sensor output based on Rotor Angle ==
  data: theta input; Ha output; Hb output; Hc output
function [Ha,Hb,Hc] = fcn(theta)

if (theta>330 && theta<=360) || (theta>=0 && theta<=30)
    Ha=1;
    Hb=0;
    Hc=1;

elseif (theta>30 && theta<=90)
    Ha=1;
    Hb=0;
    Hc=0;
elseif (theta>90 && theta<=150)
    Ha=1;
    Hb=1;
    Hc=0;
elseif (theta>150 && theta<=210)
    Ha=0;
    Hb=1;
    Hc=0;
elseif (theta>210 && theta<=270)
    Ha=0;
    Hb=1;
    Hc=1;
elseif (theta>270 && theta<=330)
    Ha=0;
    Hb=0;
    Hc=1;
else
    Ha=0;
    Hb=0;
    Hc=0;
end

== matlab function Five_level_MCI_PMSM_Control_1_fault_tolerant/Controller/MATLAB Function1 ==
  data: L input; G1 output; G2 output; G3 output; G4 output; G5 output; G6 output; G7 output; G8 output
function [G1,G2,G3,G4,G5,G6,G7,G8] = CHB5_Gating(L)
%#codegen
% Input: L ∈ {-2, -1, 0, 1, 2}
% Output: 8 gate signals (4 per H-bridge, total 2 bridges)

% Initialize all gate signals
G1=0; G2=0; G3=0; G4=0;
G5=0; G6=0; G7=0; G8=0;

switch L
    case 2   % +2Vdc = +Vdc + +Vdc
        [G1,G2,G3,G4] = deal(1,1,0,0);  % Bridge 1: +Vdc
        [G5,G6,G7,G8] = deal(1,1,0,0);  % Bridge 2: +Vdc
        
    case 1   % +Vdc = +Vdc + 0
        [G1,G2,G3,G4] = deal(1,1,0,0);  % Bridge 1: +Vdc
        [G5,G6,G7,G8] = deal(0,1,1,0);  % Bridge 2: 0
        
    case 0   % 0 = 0 + 0
        [G1,G2,G3,G4] = deal(0,1,1,0);  % Bridge 1: 0
        [G5,G6,G7,G8] = deal(0,1,1,0);  % Bridge 2: 0
        
    case -1  % -Vdc = -Vdc + 0
        [G1,G2,G3,G4] = deal(0,0,1,1);  % Bridge 1: -Vdc
        [G5,G6,G7,G8] = deal(0,1,1,0);  % Bridge 2: 0
        
    case -2  % -2Vdc = -Vdc + -Vdc
        [G1,G2,G3,G4] = deal(0,0,1,1);  % Bridge 1: -Vdc
        [G5,G6,G7,G8] = deal(0,0,1,1);  % Bridge 2: -Vdc
end
end

== matlab function Five_level_MCI_PMSM_Control_1_fault_tolerant/Controller/MATLAB Function2 ==
  data: L input; G1 output; G2 output; G3 output; G4 output; G5 output; G6 output; G7 output; G8 output
function [G1,G2,G3,G4,G5,G6,G7,G8] = CHB5_Gating(L)
%#codegen
% Input: L ∈ {-2, -1, 0, 1, 2}
% Output: 8 gate signals (4 per H-bridge, total 2 bridges)

% Initialize all gate signals
G1=0; G2=0; G3=0; G4=0;
G5=0; G6=0; G7=0; G8=0;

switch L
    case 2   % +2Vdc = +Vdc + +Vdc
        [G1,G2,G3,G4] = deal(1,1,0,0);  % Bridge 1: +Vdc
        [G5,G6,G7,G8] = deal(1,1,0,0);  % Bridge 2: +Vdc
        
    case 1   % +Vdc = +Vdc + 0
        [G1,G2,G3,G4] = deal(1,1,0,0);  % Bridge 1: +Vdc
        [G5,G6,G7,G8] = deal(0,1,1,0);  % Bridge 2: 0
        
    case 0   % 0 = 0 + 0
        [G1,G2,G3,G4] = deal(0,1,1,0);  % Bridge 1: 0
        [G5,G6,G7,G8] = deal(0,1,1,0);  % Bridge 2: 0
        
    case -1  % -Vdc = -Vdc + 0
        [G1,G2,G3,G4] = deal(0,0,1,1);  % Bridge 1: -Vdc
        [G5,G6,G7,G8] = deal(0,1,1,0);  % Bridge 2: 0
        
    case -2  % -2Vdc = -Vdc + -Vdc
        [G1,G2,G3,G4] = deal(0,0,1,1);  % Bridge 1: -Vdc
        [G5,G6,G7,G8] = deal(0,0,1,1);  % Bridge 2: -Vdc
end
end

== matlab function Five_level_MCI_PMSM_Control_1_fault_tolerant/Controller/MATLAB Function3 ==
  data: L input; G1 output; G2 output; G3 output; G4 output; G5 output; G6 output; G7 output; G8 output
function [G1,G2,G3,G4,G5,G6,G7,G8] = CHB5_Gating(L)
%#codegen
% Input: L ∈ {-2, -1, 0, 1, 2}
% Output: 8 gate signals (4 per H-bridge, total 2 bridges)

% Initialize all gate signals
G1=0; G2=0; G3=0; G4=0;
G5=0; G6=0; G7=0; G8=0;

switch L
    case 2   % +2Vdc = +Vdc + +Vdc
        [G1,G2,G3,G4] = deal(1,1,0,0);  % Bridge 1: +Vdc
        [G5,G6,G7,G8] = deal(1,1,0,0);  % Bridge 2: +Vdc
        
    case 1   % +Vdc = +Vdc + 0
        [G1,G2,G3,G4] = deal(1,1,0,0);  % Bridge 1: +Vdc
        [G5,G6,G7,G8] = deal(0,1,1,0);  % Bridge 2: 0
        
    case 0   % 0 = 0 + 0
        [G1,G2,G3,G4] = deal(0,1,1,0);  % Bridge 1: 0
        [G5,G6,G7,G8] = deal(0,1,1,0);  % Bridge 2: 0
        
    case -1  % -Vdc = -Vdc + 0
        [G1,G2,G3,G4] = deal(0,0,1,1);  % Bridge 1: -Vdc
        [G5,G6,G7,G8] = deal(0,1,1,0);  % Bridge 2: 0
        
    case -2  % -2Vdc = -Vdc + -Vdc
        [G1,G2,G3,G4] = deal(0,0,1,1);  % Bridge 1: -Vdc
        [G5,G6,G7,G8] = deal(0,0,1,1);  % Bridge 2: -Vdc
end
end
